simulink model "GSFR_Individual_Vars_sensitivity"  (R2019b)
settings: Solver=VariableStepAuto  StartTime=0  StopTime=20.0  MaxStep=0.01  RelTol=1e-3
values from neighbouring files (symbols this model uses):
  D = (1*(Accuracy/100))*randn()+1    [idek.m]    (also in sensitivity_Analysis_H.m = 1; sensitivity_Analysis_R.m = (Var_Mean*(Accuracy/100))*randn()+Var_Mean; sensitivity_Analysis_pd.m = 1)
  Fh = (0.3*(Accuracy/100))*randn()+0.3    [idek.m]    (also in sensitivity_Analysis_H.m = 0.25; sensitivity_Analysis_R.m = 0.3; sensitivity_Analysis_pd.m = 0.25)
  H = (4*(Accuracy/100))*randn()+4    [idek.m]    (also in sensitivity_Analysis_H.m = (H_Mean*(Accuracy/100))*randn()+H_Mean; sensitivity_Analysis_R.m = 4; sensitivity_Analysis_pd.m = 4)
  K = (0.95*(Accuracy/100))*randn()+0.95    [idek.m]    (also in sensitivity_Analysis_H.m = 0.95; sensitivity_Analysis_R.m = 0.95; sensitivity_Analysis_pd.m = 0.95)
  R = (0.05*(Accuracy/100))*randn()+0.05    [idek.m]    (also in sensitivity_Analysis_H.m = 0.075; sensitivity_Analysis_R.m = 0.075; sensitivity_Analysis_pd.m = 0.075)
  Tr = (8*(Accuracy/100))*randn()+8    [idek.m]    (also in sensitivity_Analysis_H.m = 9; sensitivity_Analysis_R.m = 9; sensitivity_Analysis_pd.m = 9)
settings Model: EnablePacing=on  PacingRate=1000  OrderedModelArguments=off  Creator=ruiva  LastModifiedBy=ruiva

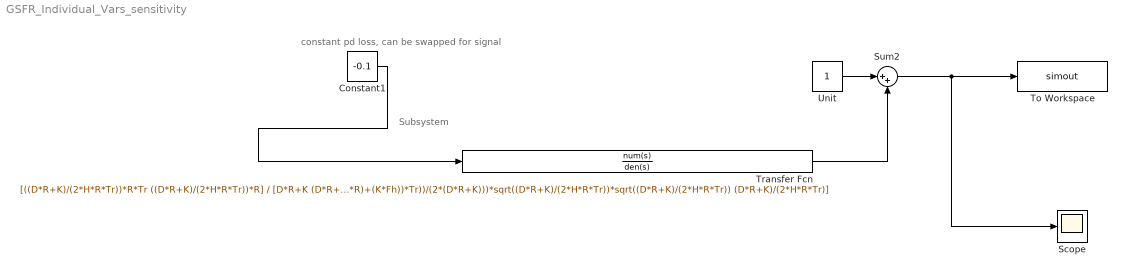
== system GSFR_Individual_Vars_sensitivity ==
  note: Subsystem
  note: constant pd loss, can be swapped for signal
  Constant1 : Constant  Value=-0.1
  Scope : Scope
  Sum2 : Sum  Inputs=|++
  To Workspace : ToWorkspace  VariableName=simout  SaveFormat=Timeseries  SampleTime=-1
  Transfer Fcn : TransferFcn  Numerator=[((D*R+K)/(2*H*R*Tr))*R*Tr ((D*R+K)/(2*H*R*Tr))*R]  Denominator=[D*R+K (D*R+K)*2*(((2*H*R)+(((D*R)+(K*Fh))*Tr))/(2*(D*R+K)))*sqrt((D*R+K)/(2*H*R*Tr))*sqrt((D*R+K)/(2*H*R*Tr)) (D*R+K)/(2*H*R*Tr)]
  Unit : Constant
  wires:
  Transfer Fcn/1 -> Sum2/2
  Unit/1 -> Sum2/1
  Sum2/1 -> Scope/1, To Workspace/1
  Constant1/1 -> Transfer Fcn/1
